simulink model "MulAdd"  (R2022b)
settings: Solver=VariableStepAuto  StartTime=0.0  StopTime=10.0  RelTol=1e-3
settings Model: Creator=Km  LastModifiedBy=Km

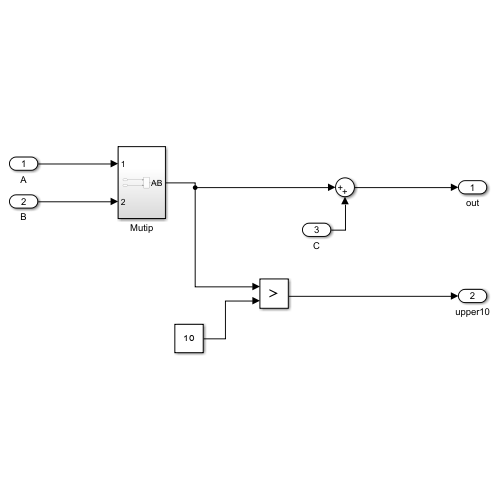
[thumbnail: Simulink's stored preview of the top-level diagram]
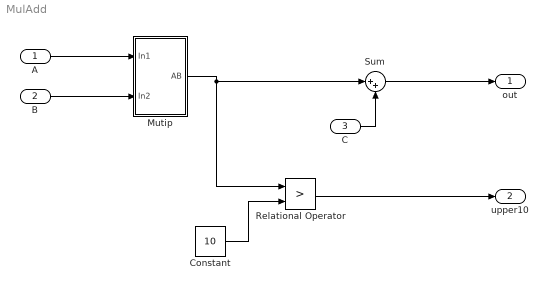
== system MulAdd ==
  A : Inport
  B : Inport  Port=2
  C : Inport  Port=3
  Constant : Constant  Value=10
  Mutip : Subsystem
  Relational Operator : RelationalOperator  Operator=>  OutDataTypeStr=boolean  RndMeth=Simplest  InputSameDT=off
  Sum : Sum  Inputs=|++
  out : Outport
  upper10 : Outport  Port=2
  wires:
  Constant/1 -> Relational Operator/2
  Sum/1 -> out/1
  C/1 -> Sum/2
  Relational Operator/1 -> upper10/1
  B/1 -> Mutip/2(In2)
  Mutip/1(AB) -> Relational Operator/1, Sum/1
  A/1 -> Mutip/1(In1)

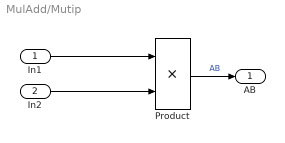
== system MulAdd/Mutip ==
  In1 : Inport
  In2 : Inport  Port=2
  Product : Product
  AB : Outport
  wires:
  In2/1 -> Product/2
  In1/1 -> Product/1
  Product/1 -> AB/1  "AB"
